simulink model "ifactionn"  (R2022b)
settings: Solver=FixedStepAuto  StartTime=0.0  StopTime=10.0  FixedStep=1e-3  RelTol=1e-3
libraries: simulink x1
settings Model: Creator=brbar  LastModifiedBy=brbar

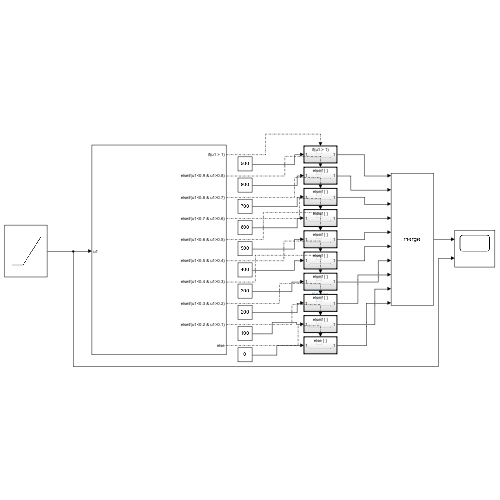
[thumbnail: Simulink's stored preview of the top-level diagram]
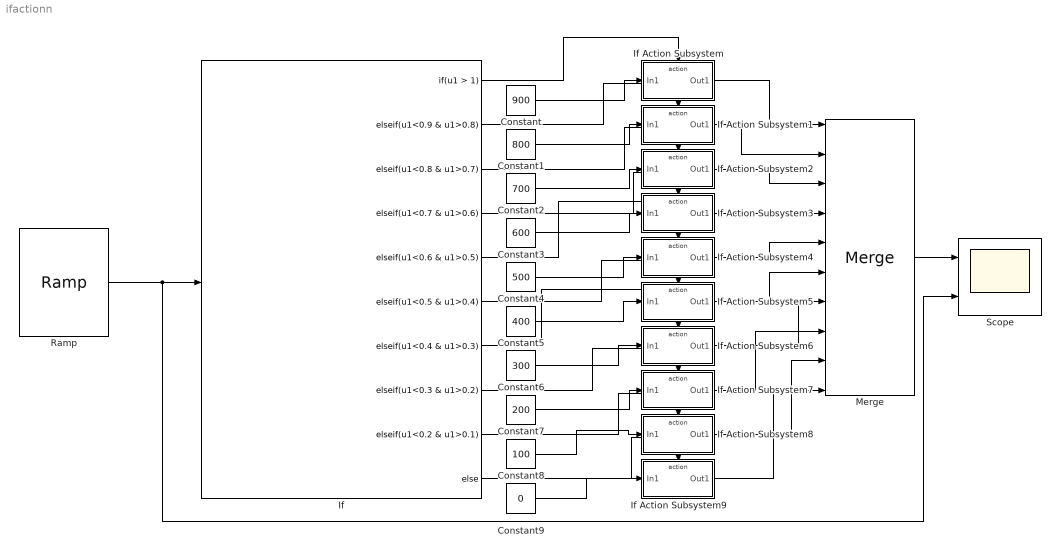
== system ifactionn ==
  Constant : Constant  Value=900
  Constant1 : Constant  Value=800
  Constant2 : Constant  Value=700
  Constant3 : Constant  Value=600
  Constant4 : Constant  Value=500
  Constant5 : Constant  Value=400
  Constant6 : Constant  Value=300
  Constant7 : Constant  Value=200
  Constant8 : Constant  Value=100
  Constant9 : Constant  Value=0
  If : If  IfExpression=u1 > 1  ElseIfExpressions=u1<0.9 & u1>0.8,u1<0.8 & u1>0.7,u1<0.7 & u1>0.6,u1<0.6 & u1>0.5,u1<0.5 & u1>0.4,u1<0.4 & u1>0.3,u1<0.3 & u1>0.2,u1<0.2 & u1>0.1
  If Action Subsystem : Subsystem  TreatAsAtomicUnit=on
  If Action Subsystem1 : Subsystem  TreatAsAtomicUnit=on
  If Action Subsystem2 : Subsystem  TreatAsAtomicUnit=on
  If Action Subsystem3 : Subsystem  TreatAsAtomicUnit=on
  If Action Subsystem4 : Subsystem  TreatAsAtomicUnit=on
  If Action Subsystem5 : Subsystem  TreatAsAtomicUnit=on
  If Action Subsystem6 : Subsystem  TreatAsAtomicUnit=on
  If Action Subsystem7 : Subsystem  TreatAsAtomicUnit=on
  If Action Subsystem8 : Subsystem  TreatAsAtomicUnit=on
  If Action Subsystem9 : Subsystem  TreatAsAtomicUnit=on
  Merge : Merge  Inputs=10
  Ramp : simulink/Sources/Ramp  slope=1  start=0  InitialOutput=0
  Scope : Scope  NumInputPorts=2
  wires:
  Ramp/1 -> Scope/2, If/1
  Merge/1 -> Scope/1
  If/1 -> If Action Subsystem/Action
  If/2 -> If Action Subsystem1/Action
  If/3 -> If Action Subsystem2/Action
  If/4 -> If Action Subsystem3/Action
  If/5 -> If Action Subsystem4/Action
  If/6 -> If Action Subsystem5/Action
  If/7 -> If Action Subsystem6/Action
  If/8 -> If Action Subsystem7/Action
  If/9 -> If Action Subsystem8/Action
  If/10 -> If Action Subsystem9/Action
  Constant/1 -> If Action Subsystem/1(In1)
  Constant1/1 -> If Action Subsystem1/1(In1)
  Constant2/1 -> If Action Subsystem2/1(In1)
  Constant3/1 -> If Action Subsystem3/1(In1)
  Constant4/1 -> If Action Subsystem4/1(In1)
  Constant5/1 -> If Action Subsystem5/1(In1)
  Constant6/1 -> If Action Subsystem6/1(In1)
  Constant7/1 -> If Action Subsystem7/1(In1)
  Constant8/1 -> If Action Subsystem8/1(In1)
  Constant9/1 -> If Action Subsystem9/1(In1)
  If Action Subsystem/1(Out1) -> Merge/1
  If Action Subsystem1/1(Out1) -> Merge/2
  If Action Subsystem2/1(Out1) -> Merge/3
  If Action Subsystem3/1(Out1) -> Merge/4
  If Action Subsystem4/1(Out1) -> Merge/5
  If Action Subsystem5/1(Out1) -> Merge/6
  If Action Subsystem6/1(Out1) -> Merge/7
  If Action Subsystem7/1(Out1) -> Merge/8
  If Action Subsystem8/1(Out1) -> Merge/9
  If Action Subsystem9/1(Out1) -> Merge/10

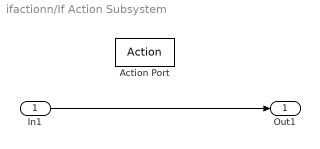
== system ifactionn/If Action Subsystem ==
  In1 : Inport
  Action Port : ActionPort  ActionPortLabel=if(u1 > 1)
  Out1 : Outport
  wires:
  In1/1 -> Out1/1

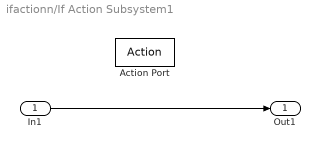
== system ifactionn/If Action Subsystem1 ==
  In1 : Inport
  Action Port : ActionPort  ActionPortLabel=elseif(u1<0.9 & u1>0.8)
  Out1 : Outport
  wires:
  In1/1 -> Out1/1

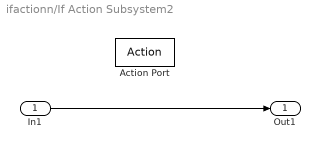
== system ifactionn/If Action Subsystem2 ==
  In1 : Inport
  Action Port : ActionPort  ActionPortLabel=elseif(u1<0.8 & u1>0.7)
  Out1 : Outport
  wires:
  In1/1 -> Out1/1

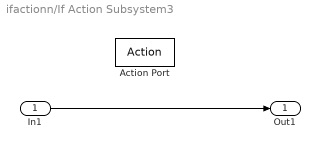
== system ifactionn/If Action Subsystem3 ==
  In1 : Inport
  Action Port : ActionPort  ActionPortLabel=elseif(u1<0.7 & u1>0.6)
  Out1 : Outport
  wires:
  In1/1 -> Out1/1

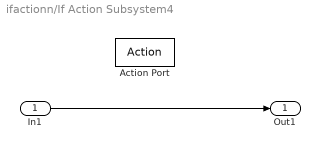
== system ifactionn/If Action Subsystem4 ==
  In1 : Inport
  Action Port : ActionPort  ActionPortLabel=elseif(u1<0.6 & u1>0.5)
  Out1 : Outport
  wires:
  In1/1 -> Out1/1

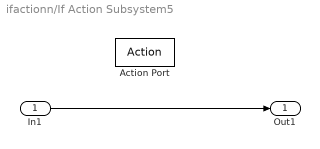
== system ifactionn/If Action Subsystem5 ==
  In1 : Inport
  Action Port : ActionPort  ActionPortLabel=elseif(u1<0.5 & u1>0.4)
  Out1 : Outport
  wires:
  In1/1 -> Out1/1

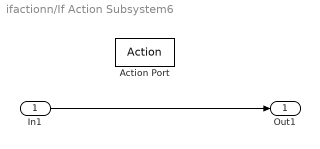
== system ifactionn/If Action Subsystem6 ==
  In1 : Inport
  Action Port : ActionPort  ActionPortLabel=elseif(u1<0.4 & u1>0.3)
  Out1 : Outport
  wires:
  In1/1 -> Out1/1

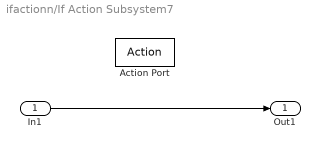
== system ifactionn/If Action Subsystem7 ==
  In1 : Inport
  Action Port : ActionPort  ActionPortLabel=elseif(u1<0.3 & u1>0.2)
  Out1 : Outport
  wires:
  In1/1 -> Out1/1

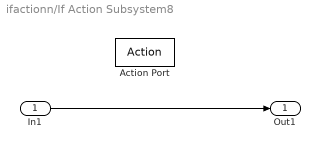
== system ifactionn/If Action Subsystem8 ==
  In1 : Inport
  Action Port : ActionPort  ActionPortLabel=elseif(u1<0.2 & u1>0.1)
  Out1 : Outport
  wires:
  In1/1 -> Out1/1

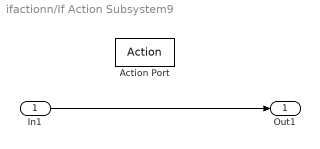
== system ifactionn/If Action Subsystem9 ==
  In1 : Inport
  Action Port : ActionPort  ActionPortLabel=else
  Out1 : Outport
  wires:
  In1/1 -> Out1/1
